simulink model "FBNREL_Ex2"  (Simulink 8.6)
settings: Solver=ode4  StartTime=0.0  StopTime=inf  FixedStep=dt  RelTol=1e-3
undefined symbols (not defined in the file): Parameter
settings Model: Creator=ivohoutzager  LastModifiedBy=schlipf  ParamWorkspaceSource=ReferencedWorkspace
settings DataIOCC: SignalLoggingSaveFormat=Dataset  SaveOutput=off  SignalLogging=off  SaveTime=off
settings OptimizationCC: DefaultParameterBehavior=Inlined
settings DebuggingCC: InheritedTsInSrcMsg=none  FcnCallInpInsideContextMsg=UseLocalSettings
settings RTWCC: SystemTargetFile=discon_grt.tlc  TemplateMakefile=discon_vc_05.tmf  Description=Bladed Style DLL  TargetLang=C++  RTWCompilerOptimization=on
settings RTWCC: CustomSource=|
  | Helpers.cpp
  | ExternalParameters.cpp
  | LegacyExternalControllerApi.cpp
settings CodeAppCC: MaxIdLength=63
settings GRTTargetCC: CombineOutputUpdateFcns=on  GRTInterface=off  UseToolchainInfoCompliant=off

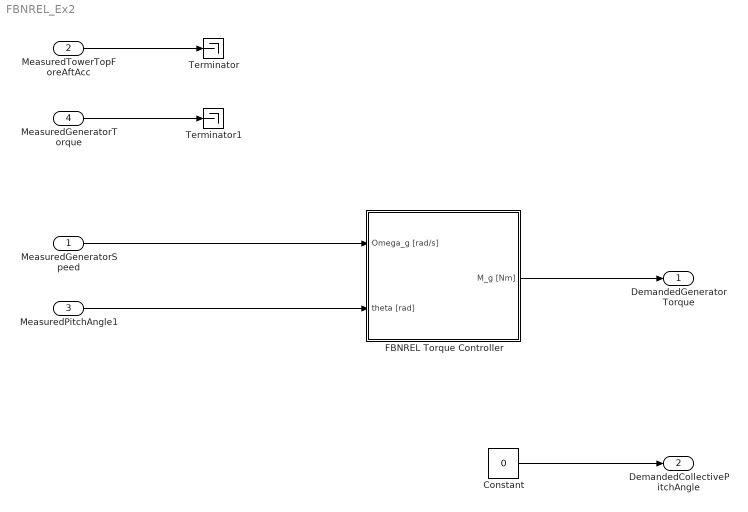
== system FBNREL_Ex2 ==
  MeasuredGeneratorSpeed : Inport  PortDimensions=1
  MeasuredTowerTopForeAftAcc : Inport  Port=2  PortDimensions=1
  MeasuredPitchAngle1 : Inport  Port=3  PortDimensions=1
  MeasuredGeneratorTorque : Inport  Port=4  PortDimensions=1
  Constant : Constant  Value=0
  FBNREL Torque Controller : Subsystem
  Terminator : Terminator
  Terminator1 : Terminator
  DemandedGeneratorTorque : Outport  PortDimensions=1
  DemandedCollectivePitchAngle : Outport  Port=2  PortDimensions=1
  wires:
  MeasuredTowerTopForeAftAcc/1 -> Terminator/1
  MeasuredGeneratorTorque/1 -> Terminator1/1
  FBNREL Torque Controller/1(M_g [Nm]) -> DemandedGeneratorTorque/1
  Constant/1 -> DemandedCollectivePitchAngle/1
  MeasuredPitchAngle1/1 -> FBNREL Torque Controller/2(theta [rad])
  MeasuredGeneratorSpeed/1 -> FBNREL Torque Controller/1(Omega_g [rad/s])

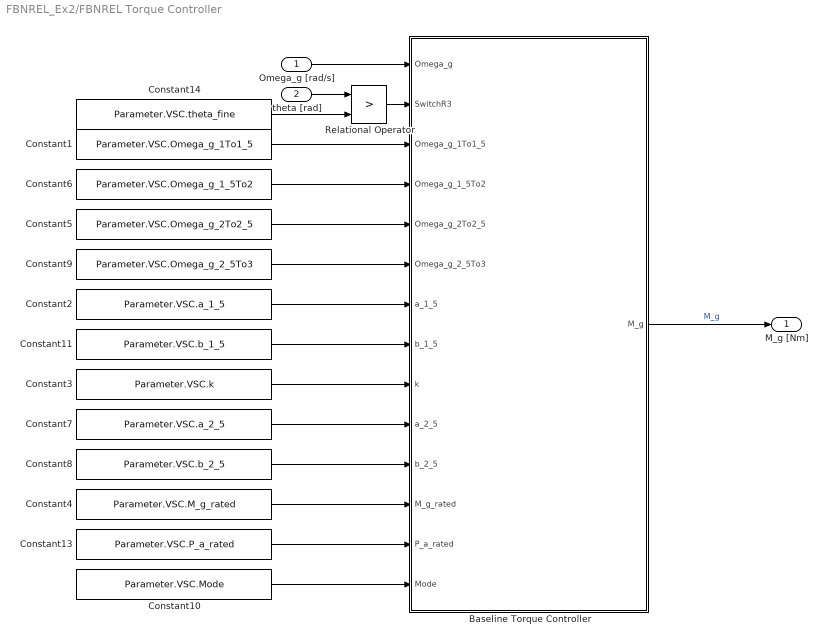
== system FBNREL_Ex2/FBNREL Torque Controller ==
  Omega_g [rad/s] : Inport
  theta [rad] : Inport  Port=2
  Baseline Torque Controller : MATLAB Function  TreatAsAtomicUnit=on
  Constant1 : Constant  Value=Parameter.VSC.Omega_g_1To1_5
  Constant10 : Constant  Value=Parameter.VSC.Mode
  Constant11 : Constant  Value=Parameter.VSC.b_1_5
  Constant13 : Constant  Value=Parameter.VSC.P_a_rated
  Constant14 : Constant  Value=Parameter.VSC.theta_fine
  Constant2 : Constant  Value=Parameter.VSC.a_1_5
  Constant3 : Constant  Value=Parameter.VSC.k
  Constant4 : Constant  Value=Parameter.VSC.M_g_rated
  Constant5 : Constant  Value=Parameter.VSC.Omega_g_2To2_5
  Constant6 : Constant  Value=Parameter.VSC.Omega_g_1_5To2
  Constant7 : Constant  Value=Parameter.VSC.a_2_5
  Constant8 : Constant  Value=Parameter.VSC.b_2_5
  Constant9 : Constant  Value=Parameter.VSC.Omega_g_2_5To3
  Relational Operator : RelationalOperator  Operator=>  OutDataTypeStr=boolean
  M_g [Nm] : Outport
  wires:
  Constant13/1 -> Baseline Torque Controller/13(P_a_rated)
  Constant11/1 -> Baseline Torque Controller/8(b_1_5)
  Constant2/1 -> Baseline Torque Controller/7(a_1_5)
  Constant10/1 -> Baseline Torque Controller/14(Mode)
  Constant3/1 -> Baseline Torque Controller/9(k)
  Constant7/1 -> Baseline Torque Controller/10(a_2_5)
  Constant8/1 -> Baseline Torque Controller/11(b_2_5)
  Constant4/1 -> Baseline Torque Controller/12(M_g_rated)
  Constant9/1 -> Baseline Torque Controller/6(Omega_g_2_5To3)
  Constant6/1 -> Baseline Torque Controller/4(Omega_g_1_5To2)
  Constant5/1 -> Baseline Torque Controller/5(Omega_g_2To2_5)
  Constant1/1 -> Baseline Torque Controller/3(Omega_g_1To1_5)
  Baseline Torque Controller/1(M_g) -> M_g [Nm]/1  "M_g"
  Omega_g [rad/s]/1 -> Baseline Torque Controller/1(Omega_g)
  Constant14/1 -> Relational Operator/2
  theta [rad]/1 -> Relational Operator/1
  Relational Operator/1 -> Baseline Torque Controller/2(SwitchR3)

== matlab function FBNREL Torque Controller/Baseline Torque Controller ==
  settings: fimath=|
      | fimath(...
      | 'RoundMode', 'floor',...
      | 'OverflowMode', 'wrap',...
      | 'ProductMode', 'KeepLSB', 'ProductWordLength', 32,...
      | 'SumMode', 'KeepLSB', 'SumWordLength', 32,...
      | 'CastBeforeSum', false)
  data: Omega_g input double; SwitchR3 input double; Omega_g_1To1_5 input double; Omega_g_1_5To2 input double; Omega_g_2To2_5 input double; Omega_g_2_5To3 input double; a_1_5 input double; b_1_5 input double; k input double; a_2_5 input double; b_2_5 input double; M_g output double; M_g_rated input double; P_a_rated input double; Mode input double
function M_g = BaselineVSControl(Omega_g,SwitchR3,...  	% signals
    Omega_g_1To1_5,Omega_g_1_5To2,...
    Omega_g_2To2_5,Omega_g_2_5To3,...                   % region limits
    a_1_5,b_1_5,...                                    	% Region 1.5 parameters
    k,...                                             	% Region   2 parameters
    a_2_5,b_2_5,...                                    	% Region 2.5 parameters
    M_g_rated,P_a_rated,Mode)                        	% Region   3 parameters

if  Mode == 1                                         	% Power constant
    M_g_3 = P_a_rated/Omega_g;
else                                                    % Torque constant
    M_g_3 = M_g_rated;
end

if      Omega_g_2_5To3  <   Omega_g                     % Region 3
    M_g     = M_g_3;

elseif  Omega_g_2To2_5  <   Omega_g                     % Region 2.5
    M_g_2_5 = a_2_5 * Omega_g + b_2_5;
    M_g     = SwitchR3*M_g_3+(1-SwitchR3)*M_g_2_5;

elseif  Omega_g_1_5To2  <   Omega_g                     % Region 2
    M_g_2   = k * Omega_g^2;
    M_g     = SwitchR3*M_g_3+(1-SwitchR3)*M_g_2;  
    
elseif  Omega_g_1To1_5  <   Omega_g                     % Region 1.5
    M_g = a_1_5 * Omega_g + b_1_5;

else                                                    % Region 1 
    M_g = 0;    
end
